simulink model "systemm"  (Simulink 7.6)
settings: Solver=ode45  StartTime=0.0  StopTime=10.0  RelTol=1e-3
undefined symbols (not defined in the file or in its folder): powericon
libraries: powerlib11 x46, powerlib x18, powerlib_extras x1
settings Model: Creator=Dr. Lotfifard  LastModifiedBy=PC  ExtModeTrigMode=oneshot  ExtModeArmWhenConnect=off
settings DataIOCC: LimitDataPoints=off
settings OptimizationCC: BlockReduction=off  BooleanDataType=off
settings DebuggingCC: SaveWithParameterizedLinksMsg=none  SignalResolutionControl=TryResolveAllWithWarning  SolverPrmCheckMsg=none  MultiTaskDSMMsg=warning  MultiTaskCondExecSysMsg=none  StrictBusMsg=None
settings HardwareCC: TargetUnknown=on
settings RTWCC: IncludeERTFirstTime=on

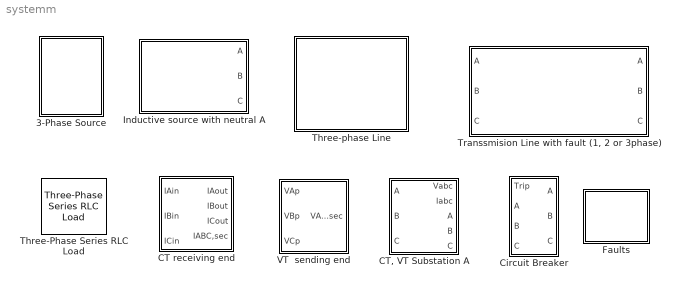
== system systemm ==
  3-Phase Source : Subsystem  mask(Three-phase Source){Vrms=1000}
      mask prompts: Vrms "RMS Voltage for each phase"
      mask Display: plot(0,0,100,100,[60,56,50,44,40,36,30,24,20],[50,40,33,40,50,60,66,60,50],[15,20,30,40,50,60,65,60,50,40,30,20,15],[50,35,27,25,26,35,50,65,73,76,73,65,50],[40,40],[90,76],[40,40],[10,25],[60,60],[75,87],[53,67],[79,79])
  CT receiving end : Subsystem  mask{TC=1.2}
      mask prompts: TC "Maximum Normal Current"
  "CT, VT Substation A" : Subsystem  mask{VT=1, CT=1}
      mask prompts: VT "VT ratio"; CT "CT ratio"
  Circuit Breaker : Subsystem
  Faults : Subsystem  mask{tof='A-G', ft=0.05, RF=1e-6}
      mask prompts: tof "Type of fault"; ft "Fault time (in sec.)"; RF "Fault Resistance RF (in ohms)"
      mask init:
      | switch tof,
      |    case 1,
      |       %No faults or Normal
      |       S1=0;S2=0;S3=0;S4=0;
      |    case 2,
      |       %Fault A-G
      |       S1=1;S2=0;S3=0;S4=1;
      |    case 3,
      |       %Fault B-G
      |       S1=0;S2=1;S3=0;S4=1;
      |    case 4,
      |       %Fault B-G
      |       S1=0;S2=0;S3=1;S4=1;
      |    case 5,
      |       %Fault B-C
      |       S1=0;S2=1;S3=1;S4=0;
      |    case 6,
      |       %Fault A-C
      |       S1=1;S2=0;S3=1;S4=0;
      |    case 7,
      |       %Fault A-B
      |       S1=1;S2=1;S3=0;S4=0;
      |    case 8,
      |       %Fault A-B-C
      |       S1=1;S2=1;S3=1;S4=0;
      |    case 9,
      |       %Fault B-C-G
      |       S1=0;S2=1;S3=1;S4=1;
      |    case 10,
      |       %Fault A-C-G
      |       S1=1;S2=0;S3=1;S4=1;
      |    case 11,
      |       %Fault A-B-G
      |       S1=1;S2=1;S3=0;S4=1;
      |    case 12,
      |       %Fault A-B-C-G
      |       S1=1;S2=1;S3=1;S4=1;
      |    end;
      mask StyleString: popup('Normal'|'A-G'|'B-G'|'C-G'|'B-C'|'A-C'|'A-B'|'A-B-C'|'B-C-G'|'A-C-G'|'A-B-G'|'A-B-C-G'),edit,edit
      mask Display: plot(0,0,100,100,[44,47,56,38,50],[23,8,64,44,97],[56,47],[25,8])
  Inductive source with neutral A : Subsystem  mask(3-phase inductive source - Ungrounded neutral){V=500000/sqrt(3)*sqrt(2), Phi=0, F=60, R=0.724, L=19.2e-3}
      mask prompts: V "Voltage magnitude (V) :"; Phi "Phase angle of phase A (Degrees) :"; F "Frequency (Hz) :"; R "Source resistance (Ohms):"; L "Source inductance (H) :"
      mask init:
      | a=R;b=L;c=inf;
      | short_x =[0,150];
      | short_y =[0,0];
      | 
      | resistor_x = [0 30,30,38,53,68,83,98,113,120,120,150];
      | resistor_y = [0,0,0,25,-25,25,-25,25,-25,0,0,0];
      | 
      | inductor_x = [150,173,173,174,178,184,190,197,202,205,206,204,201,201,197,196,198,201,207,214,220,225,229,229,227,224,224,220,219,221,225,230,237,243,249,252,253,251,247,247,244,243,244,248,254,260,267,272,275,276,276,300];
      | 
      | inductor_y = [0,0,1,11,19,24,25,23,17,8,-2,-12,-18,-18,-9,1,11,19,24,25,23,17,8,-2,-12,-18,-18,-9,1,11,19,24,25,23,17,8,-2,-12,-18,-18,-9,1, 11,19,24,25,23,17,8,0,0,0];
      | 
      | capacitor_x1 = [300 360 360 360];
      | capacitor_y1 = [0 0 25 -25];
      | capacitor_x2 = [390 390 390 450];
      | capacitor_y2 = [25,-25,0,0];
      | if a~=0
      | 	s1=resistor_x;
      | 	s2=resistor_y;
      | else
      | 	s1=short_x;
      | 	s2=short_y;
      | end
      | 
      | if b~=0
      | 	s3=inductor_x;
      | 	s4=inductor_y;
      | else
      | 	s3=short_x+150;
      | 	s4=short_y;
      | end
      | 
      | s5=[];
      | s6=[];
      | s7=[];
      | s8=[];
      mask Display: plot(-170,-60,360,60,s1,s2,s3,s4,s5,s6,s7,s8, [0,9,18,24,29,30,29,24,18,9,0,-9,-18,-24,-29,-30,-29,-24,-18,-9,0]*1.5-45,  [30,29,24,18,9,0,-9,-18,-24,-29,-30,-29,-24,-18,-9,0,9,18,24,29,30]*0.8,[-150,-90],[0,0],[-150,-150],[-20,20],[-165,-165],[-15,15],[-180,-180],[-10,10])
  Three-Phase Series RLC Load : powerlib/Elements/Three-Phase Series RLC Load  DialogController=POWERSYS.PowerSysDialog  PhysicalDomain=powersysdomain  SubClassName=unknown  LeftPortType=p1  RightPortType=p1  LConnTagsString=A|B|C  Configuration=Y (grounded)  NominalVoltage=1000  NominalFrequency=60  ActivePower=10e3  InductivePower=100  CapacitivePower=100  Measurements=None
  Three-phase Line : Subsystem  mask(Three-pase Line){KM=50}
      mask prompts: KM "Fault location (1% to 99%) (the lenght of the line is 100 km):"
      mask Display: plot(0,0,100,100,[20,20,80,80,90,80,80,20,20,10],[50,40,40,50,50,50,61,61,50,50],[56,39],[55,55],[44,44],[44,55],[53,50,50],[44,48,55])
  "Transsmision Line with fault (1, 2 or 3phase)" : Subsystem  mask(Teansmission line with fault){ff=60, rr=[0.025485 0.57504], ll=[1.5760e-3 4.5291e-3], cc=[19.1e-9 11.2e-9], length=200, faultLocation=0.1, faultType='A-G', faultR=1, faultTime=[0.034 1 1 1 1]}
      mask prompts: ff "Frequency used for R L C specification (Hz)"; rr "Resistance per unit length (Ohm/km) [R1 R0]"; ll "Inductance per unit length (H/km) [L1 L0]"; cc "Capacitance per unit length (F/km) [C1 C0]"; length "Line length (km)"; faultLocation "Fault location (p.u.) <0,1>"; faultType "Fault Type"; faultR "Fault Resistance per Phase (Ohm)"; faultTime "Fault time sequence (s) [C O C O C]"
      mask StyleString: edit,edit,edit,edit,edit,edit,popup('A-G'|'A-B'|'A-B-G'|'A-B-C'|'A-B-C-G'),edit,edit
  VT  sending end : Subsystem  mask{TP=1000}
      mask prompts: TP "Nominal Voltage,rms"

== system systemm/3-Phase Source ==
  Ground : powerlib/Elements/Ground  DialogController=POWERSYS.PowerSysDialog  PhysicalDomain=powersysdomain  SubClassName=unknown  LeftPortType=p1  RightPortType=p1  LConnTagsString=a
  Internal Impedance : powerlib/Elements/Three-Phase Parallel RLC Branch  DialogController=POWERSYS.PowerSysDialog  PhysicalDomain=powersysdomain  SubClassName=unknown  LeftPortType=p1  RightPortType=p1  LConnTagsString=A|B|C  RConnTagsString=A|B|C  BranchType=RLC  Resistance=1  Inductance=1e-3  Capacitance=1e-6  Measurements=None
  VAp : powerlib/Electrical Sources/AC Voltage Source  DialogController=POWERSYS.PowerSysDialog  SystemSampleTime=-1  Amplitude=100  Phase=0  Frequency=60  SampleTime=0  Measurements=None
  VBp : powerlib/Electrical Sources/AC Voltage Source  DialogController=POWERSYS.PowerSysDialog  SystemSampleTime=-1  Amplitude=100  Phase=0  Frequency=60  SampleTime=0  Measurements=None
  VCp : powerlib/Electrical Sources/AC Voltage Source  DialogController=POWERSYS.PowerSysDialog  SystemSampleTime=-1  Amplitude=100  Phase=0  Frequency=60  SampleTime=0  Measurements=None
  VA : PMIOPort  Port=1  Side=Right
  VB : PMIOPort  Port=2  Side=Right
  VC : PMIOPort  Port=3  Side=Right
  connections:
  VAp/LConn1 -- VCp/LConn1 -- VBp/LConn1 -- Ground/LConn1
  Internal Impedance/LConn3 -- VCp/RConn1
  Internal Impedance/LConn2 -- VBp/RConn1
  Internal Impedance/LConn1 -- VAp/RConn1
  VA/RConn1 -- Internal Impedance/RConn1
  VB/RConn1 -- Internal Impedance/RConn2
  VC/RConn1 -- Internal Impedance/RConn3

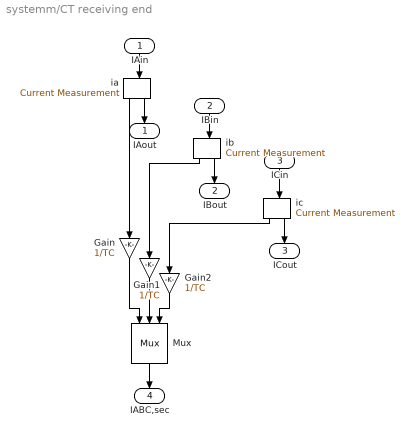
== system systemm/CT receiving end ==
  IAin : Inport
  IBin : Inport  Port=2
  ICin : Inport  Port=3
  Gain : Gain  Gain=1/TC  SaturateOnIntegerOverflow=on  OutDataTypeStr=Inherit: Same as input  ParamDataTypeStr=Inherit: Same as input
  Gain1 : Gain  Gain=1/TC  SaturateOnIntegerOverflow=on  OutDataTypeStr=Inherit: Same as input  ParamDataTypeStr=Inherit: Same as input
  Gain2 : Gain  Gain=1/TC  SaturateOnIntegerOverflow=on  OutDataTypeStr=Inherit: Same as input  ParamDataTypeStr=Inherit: Same as input
  Mux : Mux  Inputs=3
  ia : powerlib11/Measurements/Current Measurement  Tag=PoWeRsYsTeMmEaSuReMeNt
  ib : powerlib11/Measurements/Current Measurement  Tag=PoWeRsYsTeMmEaSuReMeNt
  ic : powerlib11/Measurements/Current Measurement  Tag=PoWeRsYsTeMmEaSuReMeNt
  IAout : Outport  InitialOutput=0
  IBout : Outport  Port=2  InitialOutput=0
  ICout : Outport  Port=3  InitialOutput=0
  IABC,sec : Outport  Port=4  InitialOutput=0
  wires:
  ia/1 -> Gain/1
  ib/1 -> Gain1/1
  Gain2/1 -> Mux/3
  Gain1/1 -> Mux/2
  Gain/1 -> Mux/1
  ic/1 -> Gain2/1
  IAin/1 -> ia/1
  ia/2 -> IAout/1
  IBin/1 -> ib/1
  ib/2 -> IBout/1
  ICin/1 -> ic/1
  ic/2 -> ICout/1
  Mux/1 -> IABC,sec/1

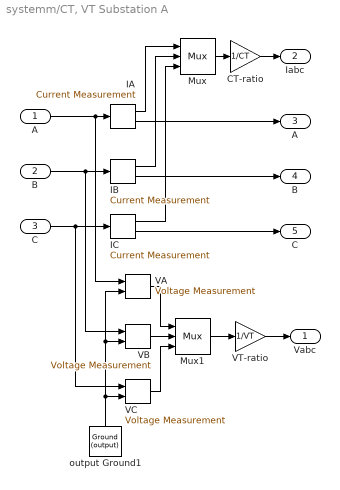
== system systemm/CT, VT Substation A ==
  A : Inport
  B : Inport  Port=2
  C : Inport  Port=3
  CT-ratio : Gain  Gain=1/CT  SaturateOnIntegerOverflow=on  OutDataTypeStr=Inherit: Same as input  ParamDataTypeStr=Inherit: Same as input
  IA : powerlib11/Measurements/Current Measurement  Tag=PoWeRsYsTeMmEaSuReMeNtFiRsT
  IB : powerlib11/Measurements/Current Measurement  Tag=PoWeRsYsTeMmEaSuReMeNt
  IC : powerlib11/Measurements/Current Measurement  Tag=PoWeRsYsTeMmEaSuReMeNt
  Mux : Mux  Inputs=3
  Mux1 : Mux  Inputs=3
  VA : powerlib11/Measurements/Voltage Measurement  Tag=PoWeRsYsTeMmEaSuReMeNt
  VB : powerlib11/Measurements/Voltage Measurement  Tag=PoWeRsYsTeMmEaSuReMeNt
  VC : powerlib11/Measurements/Voltage Measurement  Tag=PoWeRsYsTeMmEaSuReMeNt
  VT-ratio : Gain  Gain=1/VT  SaturateOnIntegerOverflow=on  OutDataTypeStr=Inherit: Same as input  ParamDataTypeStr=Inherit: Same as input
  output Ground1 : powerlib11/Connectors/Ground (output)  Tag=PoWeRsYsTeMbLoCk
  Vabc : Outport  InitialOutput=0
  Iabc : Outport  Port=2  InitialOutput=0
  " A" : Outport  Port=3  InitialOutput=0
  " B" : Outport  Port=4  InitialOutput=0
  " C" : Outport  Port=5  InitialOutput=0
  wires:
  A/1 -> IA/1, VA/1
  B/1 -> IB/1, VB/1
  C/1 -> IC/1, VC/1
  output Ground1/1 -> VC/2, VA/2, VB/2
  VA/1 -> Mux1/1
  VB/1 -> Mux1/2
  VC/1 -> Mux1/3
  IA/2 -> " A"/1
  IB/2 -> " B"/1
  IC/2 -> " C"/1
  IC/1 -> Mux/3
  IB/1 -> Mux/2
  IA/1 -> Mux/1
  Mux1/1 -> VT-ratio/1
  VT-ratio/1 -> Vabc/1
  Mux/1 -> CT-ratio/1
  CT-ratio/1 -> Iabc/1

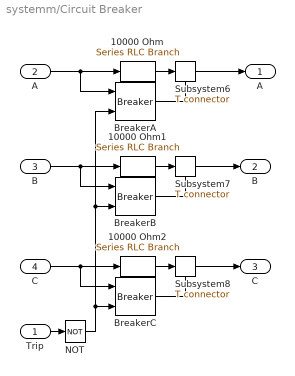
== system systemm/Circuit Breaker ==
  Trip : Inport
  A : Inport  Port=2
  B : Inport  Port=3
  C : Inport  Port=4
  10000 Ohm : powerlib11/Elements/Series RLC Branch  Tag=PoWeRsYsTeMbLoCk  a=10000  b=0  c=inf
  10000 Ohm1 : powerlib11/Elements/Series RLC Branch  Tag=PoWeRsYsTeMbLoCk  a=10000  b=0  c=inf
  10000 Ohm2 : powerlib11/Elements/Series RLC Branch  Tag=PoWeRsYsTeMbLoCk  a=10000  b=0  c=inf
  BreakerA : powerlib11/Elements/Breaker  Tag=PoWeRsYsTeMbLoCk  a=0.01  b=10e-6  c=1
  BreakerB : powerlib11/Elements/Breaker  Tag=PoWeRsYsTeMbLoCk  a=0.01  b=10e-6  c=1
  BreakerC : powerlib11/Elements/Breaker  Tag=PoWeRsYsTeMbLoCk  a=0.01  b=10e-6  c=1
  NOT : Logic  Operator=NOT  Inputs=1
  Subsystem6 : powerlib11/Connectors/T connector  Tag=PoWeRsYsTeMbLoCk
  Subsystem7 : powerlib11/Connectors/T connector  Tag=PoWeRsYsTeMbLoCk
  Subsystem8 : powerlib11/Connectors/T connector  Tag=PoWeRsYsTeMbLoCk
  " A" : Outport  InitialOutput=0
  " B" : Outport  Port=2  InitialOutput=0
  " C" : Outport  Port=3  InitialOutput=0
  wires:
  BreakerB/1 -> Subsystem7/Enable
  BreakerC/1 -> Subsystem8/Enable
  Subsystem8/1 -> " C"/1
  Subsystem7/1 -> " B"/1
  10000 Ohm1/1 -> Subsystem7/1
  BreakerA/1 -> Subsystem6/Enable
  Subsystem6/1 -> " A"/1
  C/1 -> BreakerC/1, 10000 Ohm2/1
  B/1 -> BreakerB/1, 10000 Ohm1/1
  A/1 -> BreakerA/1, 10000 Ohm/1
  10000 Ohm2/1 -> Subsystem8/1
  10000 Ohm/1 -> Subsystem6/1
  Trip/1 -> NOT/1
  NOT/1 -> BreakerC/2, BreakerB/2, BreakerA/2

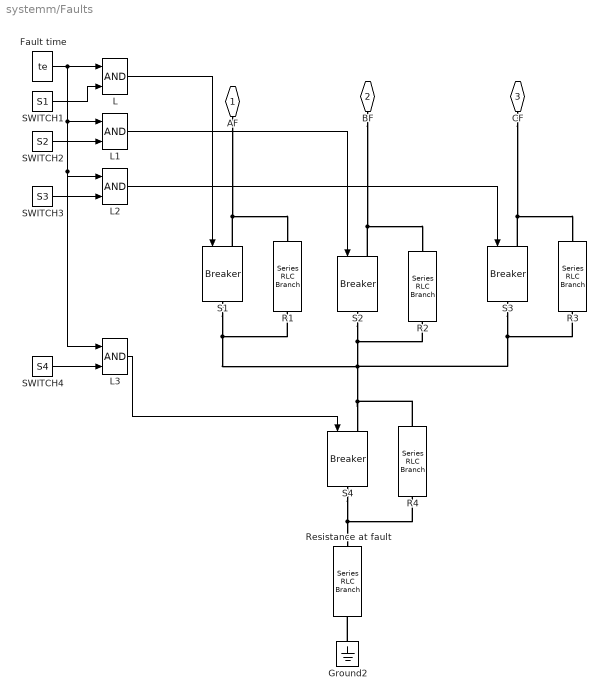
== system systemm/Faults ==
  Fault time : FromWorkspace  VariableName=te  SampleTime=0  mask( Fault timing){ t=[0 ft 10],  e=[0 1 0 ]}
      mask prompts:  t "transition steps:";  e "states (0/1):"
      mask help: steps
      mask init:
      | te=[t,t(2:length(t))-1e-8,t(length(t))+1e-8;e,e]';[y,i]=sort(te(:,1));te=[te(i,1),te(i,2)];
      mask Display: plot(te(:,1),te(:,2))
  Ground2 : powerlib/Elements/Ground  DialogController=POWERSYS.PowerSysDialog  PhysicalDomain=powersysdomain  SubClassName=unknown  LeftPortType=p1  RightPortType=p1  LConnTagsString=a
  L{,1..3} (4 alike) : Logic
  R{1..4} (4 alike) : powerlib/Elements/Series RLC Branch  DialogController=POWERSYS.PowerSysDialog  PhysicalDomain=powersysdomain  SubClassName=unknown  LeftPortType=p1  RightPortType=p1  LConnTagsString=__new0  RConnTagsString=__new0  BranchType=R  Resistance=100e6  Inductance=1e-3  SetiL0=off  InitialCurrent=0  Capacitance=1e-6  Setx0=off  InitialVoltage=0  Measurements=None
  Resistance at fault : powerlib/Elements/Series RLC Branch  DialogController=POWERSYS.PowerSysDialog  PhysicalDomain=powersysdomain  SubClassName=unknown  LeftPortType=p1  RightPortType=p1  LConnTagsString=__new0  RConnTagsString=__new0  BranchType=R  Resistance=RF  Inductance=1e-3  SetiL0=off  InitialCurrent=0  Capacitance=1e-6  Setx0=off  InitialVoltage=0  Measurements=None
  S{1..4} (4 alike) : powerlib/Elements/Breaker  DialogController=POWERSYS.PowerSysDialog  SystemSampleTime=-1  BreakerResistance=0.01  InitialState=0  SnubberResistance=1e6  SnubberCapacitance=inf  SwitchingTimes="[ 1/60  5/60 ]"  External=on  Measurements=None  MoreParameters=off  NoBreakLoop=off
  SWITCH1 : Constant  Value=S1
  SWITCH2 : Constant  Value=S2
  SWITCH3 : Constant  Value=S3
  SWITCH4 : Constant  Value=S4
  AF : PMIOPort  Port=1  Side=Left
  BF : PMIOPort  Port=2  Side=Left
  CF : PMIOPort  Port=3  Side=Left
  wires:
  Fault time/1 -> L/1, L1/1, L2/1, L3/1
  SWITCH1/1 -> L/2
  SWITCH2/1 -> L1/2
  SWITCH3/1 -> L2/2
  L/1 -> S1/1
  SWITCH4/1 -> L3/2
  L1/1 -> S2/1
  L2/1 -> S3/1
  L3/1 -> S4/1
  connections:
  S1/LConn1 -- R1/RConn1 -- AF/RConn1
  BF/RConn1 -- S2/LConn1 -- R2/RConn1
  CF/RConn1 -- S3/LConn1 -- R3/RConn1
  S1/RConn1 -- S2/RConn1 -- R2/LConn1 -- R4/RConn1 -- S4/LConn1 -- S3/RConn1 -- R3/LConn1 -- R1/LConn1
  S4/RConn1 -- R4/LConn1 -- Resistance at fault/LConn1
  Ground2/LConn1 -- Resistance at fault/RConn1

== system systemm/Inductive source with neutral A ==
  RLa : powerlib11/Elements/Series RLC Branch  Tag=PoWeRsYsTeMbLoCk  a=R  b=L  c=inf
  RLb : powerlib11/Elements/Series RLC Branch  Tag=PoWeRsYsTeMbLoCk  a=R  b=L  c=inf
  RLc : powerlib11/Elements/Series RLC Branch  Tag=PoWeRsYsTeMbLoCk  a=R  b=L  c=inf
  Va : powerlib11/Electrical Sources/AC Voltage Source  Tag=PoWeRsYsTeMbLoCk  A=V  P=Phi  F=F
  Va1 : powerlib11/Electrical Sources/AC Voltage Source  Tag=PoWeRsYsTeMbLoCk  A=V  P=Phi-120  F=F
  Va2 : powerlib11/Electrical Sources/AC Voltage Source  Tag=PoWeRsYsTeMbLoCk  A=V  P=Phi+120  F=F
  output Ground1 : powerlib11/Connectors/Ground (output)  Tag=PoWeRsYsTeMbLoCk
  A : Outport  InitialOutput=0
  B : Outport  Port=2  InitialOutput=0
  C : Outport  Port=3  InitialOutput=0
  wires:
  Va/1 -> RLa/1
  RLa/1 -> A/1
  Va1/1 -> RLb/1
  RLb/1 -> B/1
  Va2/1 -> RLc/1
  RLc/1 -> C/1
  output Ground1/1 -> Va1/1, Va/1, Va2/1

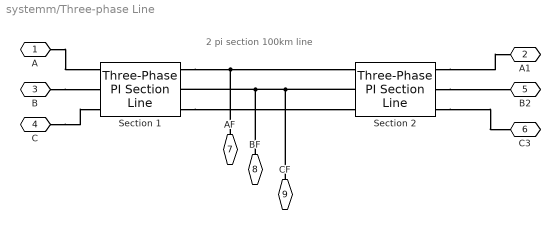
== system systemm/Three-phase Line ==
  note: 2 pi section 100km line
  Section 1 : powerlib/Elements/Three-Phase PI Section Line  DialogController=POWERSYS.PowerSysDialog  PhysicalDomain=powersysdomain  SubClassName=unknown  LeftPortType=p1  RightPortType=p1  LConnTagsString=a|b|c  RConnTagsString=A|B|C  Frequency=60  Resistances=[0.01273 0.3864]  Inductances="[0.9337e-3  4.1264e-3]"  Capacitances=[12.74e-9 7.751e-9]  Length=100
  Section 2 : powerlib/Elements/Three-Phase PI Section Line  DialogController=POWERSYS.PowerSysDialog  PhysicalDomain=powersysdomain  SubClassName=unknown  LeftPortType=p1  RightPortType=p1  LConnTagsString=a|b|c  RConnTagsString=A|B|C  Frequency=60  Resistances=[0.01273 0.3864]  Inductances="[0.9337e-3  4.1264e-3]"  Capacitances=[12.74e-9 7.751e-9]  Length=100
  A : PMIOPort  Port=1  Side=Left
  A1 : PMIOPort  Port=2  Side=Right
  B : PMIOPort  Port=3  Side=Left
  C : PMIOPort  Port=4  Side=Left
  B2 : PMIOPort  Port=5  Side=Right
  C3 : PMIOPort  Port=6  Side=Right
  AF : PMIOPort  Port=7  Side=Right
  BF : PMIOPort  Port=8  Side=Right
  CF : PMIOPort  Port=9  Side=Right
  connections:
  Section 2/RConn1 -- A1/RConn1
  Section 2/RConn2 -- B2/RConn1
  Section 2/RConn3 -- C3/RConn1
  Section 1/RConn1 -- Section 2/LConn1 -- AF/RConn1
  Section 2/LConn2 -- Section 1/RConn2 -- BF/RConn1 -- CF/RConn1
  Section 1/RConn3 -- Section 2/LConn3
  A/RConn1 -- Section 1/LConn1
  B/RConn1 -- Section 1/LConn2
  C/RConn1 -- Section 1/LConn3

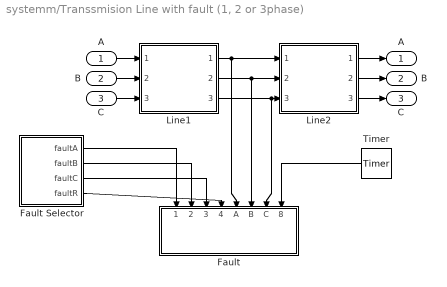
== system systemm/Transsmision Line with fault (1, 2 or 3phase) ==
  A : Inport
  B : Inport  Port=2
  C : Inport  Port=3
  Fault : Subsystem
  Fault Selector : Subsystem
  Line1 : Subsystem  Tag=PoWeRsYsTeMbLoCk  InitFcn=powericon('checksum',bdroot)  mask(Distributed Parameters Line){n=3, f=ff, r=rr, l=ll, c=cc, lgt=length*(faultLocation+0.0005)}
      mask prompts: n "Number of phases N"; f "Frequency used for R L C specification (Hz)"; r "Resistance per unit length (Ohms/km)   [N*N matrix] or [R1 R0 R0m]"; l "Inductance per unit length (H/km) [N*N matrix ] or [L1 L0 L0m]"; c "Capacitance per unit length (F/km) [N*N matrix] or [C1 C0 C0m]"; lgt "Line length (km)"
      mask help:
      | Implements a N-phases distributed parameter line model. The R,L, and C line parameters are specified by [NxN] matrices.
      |
      | To model a two-, three-, or a six-phase symetrical line you can either specify complete [NxN] matrices or simply enter sequence parameters vectors: the  positive and zero sequence parameters for a two-phase or  three-phase transposed  line, plus the mutual zero-sequence for a  six-phase transposed  line  (2 coupled 3-phase lines).
      mask init:
      | [a1,a2,a3,a4,a5,a6,gx,gy]=powericon(n,f,r,l,c);
      mask Display: plot(a1,a2,a3,a4,a5,a6,gx,gy,-10,0,110,120)
  Line2 : Subsystem  Tag=PoWeRsYsTeMbLoCk  InitFcn=powericon('checksum',bdroot)  mask(Distributed Parameters Line){n=3, f=ff, r=rr, l=ll, c=cc, lgt=length*(1-faultLocation-0.0005)}
      mask prompts: n "Number of phases N"; f "Frequency used for R L C specification (Hz)"; r "Resistance per unit length (Ohms/km)   [N*N matrix] or [R1 R0 R0m]"; l "Inductance per unit length (H/km) [N*N matrix ] or [L1 L0 L0m]"; c "Capacitance per unit length (F/km) [N*N matrix] or [C1 C0 C0m]"; lgt "Line length (km)"
      mask help:
      | Implements a N-phases distributed parameter line model. The R,L, and C line parameters are specified by [NxN] matrices.
      |
      | To model a two-, three-, or a six-phase symetrical line you can either specify complete [NxN] matrices or simply enter sequence parameters vectors: the  positive and zero sequence parameters for a two-phase or  three-phase transposed  line, plus the mutual zero-sequence for a  six-phase transposed  line  (2 coupled 3-phase lines).
      mask init:
      | [a1,a2,a3,a4,a5,a6,gx,gy]=powericon(n,f,r,l,c);
      mask Display: plot(a1,a2,a3,a4,a5,a6,gx,gy,-10,0,110,120)
  Timer : powerlib_extras/Control  Blocks/Timer  t=[0 faultTime]  e=[0 1 0 1 0 1]
  "A " : Outport  InitialOutput=0
  "B " : Outport  Port=2  InitialOutput=0
  "C " : Outport  Port=3  InitialOutput=0
  wires:
  Line1/1(" 1") -> Line2/1(1), Fault/5(A)
  Line1/2(" 2") -> Line2/2(2), Fault/6(B)
  Line1/3(" 3") -> Line2/3(3), Fault/7(C)
  Timer/1 -> Fault/8(Tfault)
  Line2/1(" 1") -> "A "/1
  A/1 -> Line1/1(1)
  Line2/2(" 2") -> "B "/1
  B/1 -> Line1/2(2)
  Line2/3(" 3") -> "C "/1
  C/1 -> Line1/3(3)
  Fault Selector/4(faultR) -> Fault/4(faultG)
  Fault Selector/3(faultC) -> Fault/3(faultC)
  Fault Selector/2(faultB) -> Fault/2(faultB)
  Fault Selector/1(faultA) -> Fault/1(faultA)

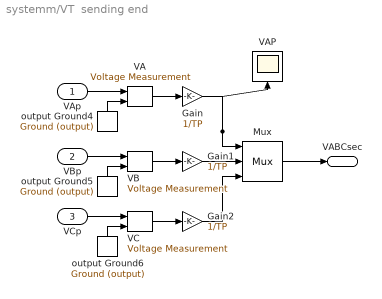
== system systemm/VT  sending end ==
  VAp : Inport
  VBp : Inport  Port=2
  VCp : Inport  Port=3
  Gain : Gain  Gain=1/TP  SaturateOnIntegerOverflow=on  OutDataTypeStr=Inherit: Same as input  ParamDataTypeStr=Inherit: Same as input
  Gain1 : Gain  Gain=1/TP  SaturateOnIntegerOverflow=on  OutDataTypeStr=Inherit: Same as input  ParamDataTypeStr=Inherit: Same as input
  Gain2 : Gain  Gain=1/TP  SaturateOnIntegerOverflow=on  OutDataTypeStr=Inherit: Same as input  ParamDataTypeStr=Inherit: Same as input
  Mux : Mux  Inputs=3
  VA : powerlib11/Measurements/Voltage Measurement  Tag=PoWeRsYsTeMmEaSuReMeNtFiRsT
  VAP : Scope
      settings: TickLabels=on  YMin=-1.5  YMax=1.75  DataFormat=Array
  VB : powerlib11/Measurements/Voltage Measurement  Tag=PoWeRsYsTeMmEaSuReMeNtFiRsT
  VC : powerlib11/Measurements/Voltage Measurement  Tag=PoWeRsYsTeMmEaSuReMeNtFiRsT
  output Ground4 : powerlib11/Connectors/Ground (output)  Tag=PoWeRsYsTeMbLoCk
  output Ground5 : powerlib11/Connectors/Ground (output)  Tag=PoWeRsYsTeMbLoCk
  output Ground6 : powerlib11/Connectors/Ground (output)  Tag=PoWeRsYsTeMbLoCk
  VABCsec : Outport
  wires:
  output Ground5/1 -> VB/2
  VBp/1 -> VB/1
  Gain1/1 -> Mux/2
  VB/1 -> Gain1/1
  Mux/1 -> VABCsec/1
  output Ground6/1 -> VC/2
  VCp/1 -> VC/1
  Gain2/1 -> Mux/3
  VC/1 -> Gain2/1
  output Ground4/1 -> VA/2
  VAp/1 -> VA/1
  VA/1 -> Gain/1
  Gain/1 -> Mux/1, VAP/1

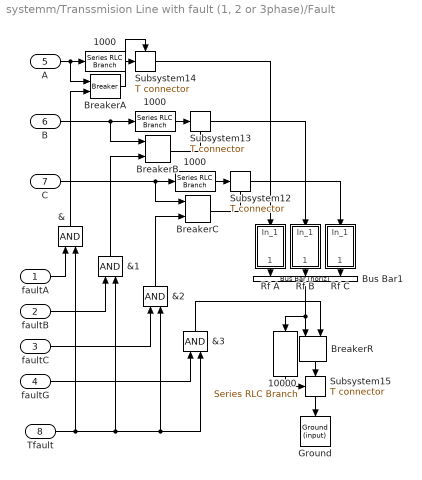
== system systemm/Transsmision Line with fault (1, 2 or 3phase)/Fault ==
  faultA : Inport
  faultB : Inport  Port=2
  faultC : Inport  Port=3
  faultG : Inport  Port=4
  A : Inport  Port=5
  B : Inport  Port=6
  C : Inport  Port=7
  Tfault : Inport  Port=8
  " 10000" : powerlib11/Elements/Series RLC Branch  Tag=PoWeRsYsTeMbLoCk  a=1000  b=0  c=inf
  &{,1..3} (4 alike) : Logic
  1000 : powerlib11/Elements/Series RLC Branch  Tag=PoWeRsYsTeMbLoCk  a=1000  b=0  c=inf
  "1000 " : powerlib11/Elements/Series RLC Branch  Tag=PoWeRsYsTeMbLoCk  a=1000  b=0  c=inf
  "1000  " : powerlib11/Elements/Series RLC Branch  Tag=PoWeRsYsTeMbLoCk  a=1000  b=0  c=inf
  BreakerA : powerlib11/Elements/Breaker  Tag=PoWeRsYsTeMbLoCk  a=0.01  b=10e-6  c=0
  BreakerB : powerlib11/Elements/Breaker  Tag=PoWeRsYsTeMbLoCk  a=0.01  b=10e-6  c=0
  BreakerC : powerlib11/Elements/Breaker  Tag=PoWeRsYsTeMbLoCk  a=0.01  b=10e-6  c=0
  BreakerR : powerlib11/Elements/Breaker  Tag=PoWeRsYsTeMbLoCk  a=0.01  b=10e-6  c=0
  Bus Bar1 : powerlib11/Connectors/Bus Bar (horiz)  Tag=PoWeRsYsTeMbLoCk  entrees=3  sorties=1
  Ground : powerlib11/Connectors/Ground (input)  Tag=PoWeRsYsTeMbLoCk
  Rf A : Subsystem  Tag=PoWeRsYsTeMbLoCk  InitFcn=powericon('checksum',bdroot)  mask(Series RLC Branch){a=faultR, b=0, c=inf}
      mask prompts: a "Resistance R (Ohms):"; b "Inductance L (H):"; c "Capacitance C (F):"
      mask help: Series RLC branch.
      mask init:
      | [s1,s2,s3,s4,r1,r2,l1,l2,c1,c2,c3,c4] = powericon(a,b,c);
      mask Help: web(psbhelp);
      mask Display: plot(s1,s2,s3,s4,r1,r2,l1,l2,c1,c2,c3,c4)
  Rf B : Subsystem  Tag=PoWeRsYsTeMbLoCk  InitFcn=powericon('checksum',bdroot)  mask(Series RLC Branch){a=faultR, b=0, c=inf}
      mask prompts: a "Resistance R (Ohms):"; b "Inductance L (H):"; c "Capacitance C (F):"
      mask help: Series RLC branch.
      mask init:
      | [s1,s2,s3,s4,r1,r2,l1,l2,c1,c2,c3,c4] = powericon(a,b,c);
      mask Help: web(psbhelp);
      mask Display: plot(s1,s2,s3,s4,r1,r2,l1,l2,c1,c2,c3,c4)
  Rf C : Subsystem  Tag=PoWeRsYsTeMbLoCk  InitFcn=powericon('checksum',bdroot)  mask(Series RLC Branch){a=faultR, b=0, c=inf}
      mask prompts: a "Resistance R (Ohms):"; b "Inductance L (H):"; c "Capacitance C (F):"
      mask help: Series RLC branch.
      mask init:
      | [s1,s2,s3,s4,r1,r2,l1,l2,c1,c2,c3,c4] = powericon(a,b,c);
      mask Help: web(psbhelp);
      mask Display: plot(s1,s2,s3,s4,r1,r2,l1,l2,c1,c2,c3,c4)
  Subsystem{12..15} (4 alike) : powerlib11/Connectors/T connector  Tag=PoWeRsYsTeMbLoCk
  wires:
  Rf A/1(Outport) -> Bus Bar1/1
  Rf B/1(Outport) -> Bus Bar1/2
  Rf C/1(Outport) -> Bus Bar1/3
  "1000  "/1 -> Subsystem12/1
  BreakerC/1 -> Subsystem12/Enable
  "1000 "/1 -> Subsystem13/1
  BreakerB/1 -> Subsystem13/Enable
  Subsystem12/1 -> Rf C/1(In_1)
  Subsystem13/1 -> Rf B/1(In_1)
  1000/1 -> Subsystem14/1
  BreakerA/1 -> Subsystem14/Enable
  Subsystem14/1 -> Rf A/1(In_1)
  B/1 -> "1000 "/1, BreakerB/1
  A/1 -> 1000/1, BreakerA/1
  C/1 -> "1000  "/1, BreakerC/1
  faultA/1 -> &/1
  &1/1 -> BreakerB/2
  &2/1 -> BreakerC/2
  faultB/1 -> &1/1
  faultC/1 -> &2/1
  BreakerR/1 -> Subsystem15/1
  Subsystem15/1 -> Ground/1
  " 10000"/1 -> Subsystem15/Enable
  Bus Bar1/1 -> BreakerR/1, " 10000"/1
  faultG/1 -> &3/1
  &3/1 -> BreakerR/2
  Tfault/1 -> &3/2, &2/2, &1/2, &/2
  &/1 -> BreakerA/2

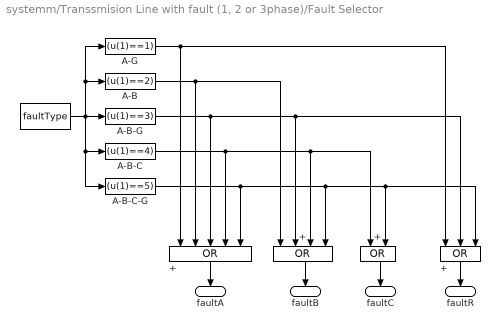
== system systemm/Transsmision Line with fault (1, 2 or 3phase)/Fault Selector ==
  "  " : Constant  Value=faultType
  "  +" : Logic  Operator=OR
  " +" : Logic  Operator=OR  Inputs=4
  + : Logic  Operator=OR  Inputs=5
  "+ " : Logic  Operator=OR  Inputs=3
  A-B : Fcn  Expr=(u(1)==2)
  A-B-C : Fcn  Expr=(u(1)==4)
  A-B-C-G : Fcn  Expr=(u(1)==5)
  A-B-G : Fcn  Expr=(u(1)==3)
  A-G : Fcn  Expr=(u(1)==1)
  faultA : Outport  InitialOutput=0
  faultB : Outport  Port=2  InitialOutput=0
  faultC : Outport  Port=3  InitialOutput=0
  faultR : Outport  Port=4  InitialOutput=0
  wires:
  "  "/1 -> A-B-G/1, A-G/1, A-B/1, A-B-C-G/1, A-B-C/1
  +/1 -> faultA/1
  " +"/1 -> faultB/1
  "  +"/1 -> faultC/1
  "+ "/1 -> faultR/1
  A-B/1 -> +/2, " +"/1
  A-B-G/1 -> +/3, " +"/2, "+ "/2
  A-B-C/1 -> +/4, " +"/3, "  +"/1
  A-B-C-G/1 -> +/5, " +"/4, "  +"/2, "+ "/3
  A-G/1 -> +/1, "+ "/1

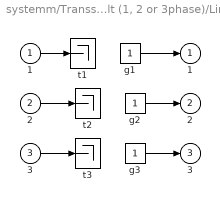
== system systemm/Transsmision Line with fault (1, 2 or 3phase)/Line1 ==
  1 : Inport
  2 : Inport  Port=2
  3 : Inport  Port=3
  g1 : Constant
  g2 : Constant
  g3 : Constant
  t1 : Terminator
  t2 : Terminator
  t3 : Terminator
  " 1" : Outport  InitialOutput=0
  " 2" : Outport  Port=2  InitialOutput=0
  " 3" : Outport  Port=3  InitialOutput=0
  wires:
  g3/1 -> " 3"/1
  3/1 -> t3/1
  g2/1 -> " 2"/1
  2/1 -> t2/1
  1/1 -> t1/1
  g1/1 -> " 1"/1

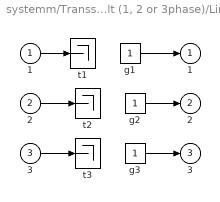
== system systemm/Transsmision Line with fault (1, 2 or 3phase)/Line2 ==
  1 : Inport
  2 : Inport  Port=2
  3 : Inport  Port=3
  g1 : Constant
  g2 : Constant
  g3 : Constant
  t1 : Terminator
  t2 : Terminator
  t3 : Terminator
  " 1" : Outport  InitialOutput=0
  " 2" : Outport  Port=2  InitialOutput=0
  " 3" : Outport  Port=3  InitialOutput=0
  wires:
  g1/1 -> " 1"/1
  1/1 -> t1/1
  2/1 -> t2/1
  g2/1 -> " 2"/1
  3/1 -> t3/1
  g3/1 -> " 3"/1

== system systemm/Transsmision Line with fault (1, 2 or 3phase)/Fault/Rf A ==
  In_1 : Inport
  Constant : Constant
  Terminator : Terminator
  Outport : Outport  InitialOutput=0
  wires:
  Constant/1 -> Outport/1
  In_1/1 -> Terminator/1

== system systemm/Transsmision Line with fault (1, 2 or 3phase)/Fault/Rf B ==
  In_1 : Inport
  Constant : Constant
  Terminator : Terminator
  Outport : Outport  InitialOutput=0
  wires:
  Constant/1 -> Outport/1
  In_1/1 -> Terminator/1

== system systemm/Transsmision Line with fault (1, 2 or 3phase)/Fault/Rf C ==
  In_1 : Inport
  Constant : Constant
  Terminator : Terminator
  Outport : Outport  InitialOutput=0
  wires:
  Constant/1 -> Outport/1
  In_1/1 -> Terminator/1
